simulink model "UDP_sensor_stream"  (R2021a)
settings: Solver=ode3  StartTime=0.0  StopTime=10.0  RelTol=1e-3
libraries: androidsensorlib x8, androidcommunicationlib x1
PreSaveFcn:
  | set_param(gcs, 'Location',[35 56 895 700 ])
settings Model: ExtModeTrigDuration=100  Creator=The MathWorks, Inc.  LastModifiedBy=shrey
settings SolverCC: AlgebraicLoopSolver=TrustRegion
settings DataIOCC: LimitDataPoints=on  SaveFormat=Array  ReturnWorkspaceOutputs=off
settings OptimizationCC: LifeSpan=1  MaxStackSize=64
settings DebuggingCC: UnderspecifiedInitializationDetection=Classic  MergeDetectMultiDrivingBlocksExec=none  ParameterPrecisionLossMsg=none  AllowSymbolicDim=off  SFUnexpectedBacktrackingDiag=warning  SFNoUnconditionalDefaultTransitionDiag=warning  SFExecutionAtInitializationDiag=none  SFMachineParentedDataDiag=warning  ArithmeticOperatorsInVariantConditions=warning
settings HardwareCC: ProdBitPerPointer=32  ProdBitPerSizeT=32  ProdBitPerPtrDiffT=32  ProdLargestAtomicInteger=Long  ProdLargestAtomicFloat=Double  ProdWordSize=32  ProdHWDeviceType=ARM Compatible->ARM Cortex  TargetLargestAtomicInteger=Long  TargetLargestAtomicFloat=Double  TargetEndianess=LittleEndian  TargetHWDeviceType=ARM Compatible->ARM Cortex  UseEmbeddedCoderFeatures=off  UseSimulinkCoderFeatures=off
settings ModelReferenceCC: PropagateSignalLabelsOutOfModel=off
settings SFSimCC: SimUseLocalCustomCode=off  CustomCodeUndefinedFunction=UseInterfaceOnly
settings RTWCC: SystemTargetFile=ert.tlc  HardwareBoard=Android Device  TemplateMakefile=ert_default_tmf  GenerateReport=on  RTWVerbose=off  RTWUseLocalCustomCode=off  Toolchain=Android SDK/NDK Tools  LaunchReport=on
settings CodeAppCC: ForceParamTrailComments=on  OperatorAnnotations=on  StateflowObjectComments=on  MATLABSourceComments=on
settings ERTTargetCC: MultiwordLength=2048  ERTCustomFileBanners=off  SupportContinuousTime=on  SupportNonInlinedSFcns=on  RemoveResetFunc=off  ModelStepFunctionPrototypeControlCompliant=off
settings ConfigComp: CovMetricSettings=dw  CovSaveCumulativeToWorkspaceVar=on  CovSaveSingleToWorkspaceVar=on  CovExternalEMLEnable=off  CovSFcnEnable=off

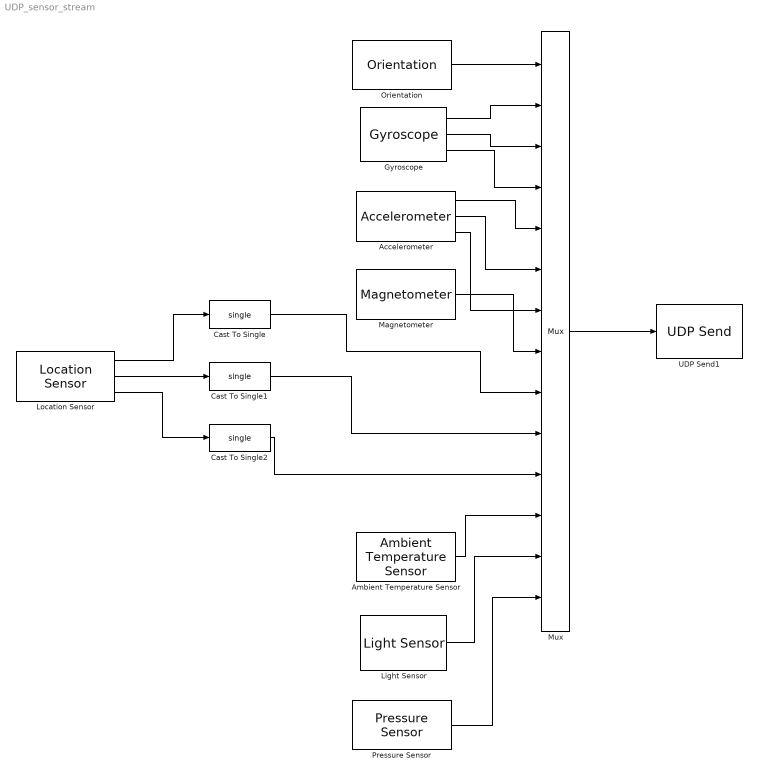
== system UDP_sensor_stream ==
  Accelerometer : androidsensorlib/Accelerometer  OutputVector=off  SampleTime=0.1  BlockPlatform=Android
      settings: SourceProductBaseCode=ANDROID
  Ambient Temperature Sensor : androidsensorlib/Ambient Temperature Sensor  SampleTime=0.1  BlockPlatform=Android
      settings: SourceProductBaseCode=ANDROID
  Cast To Single : DataTypeConversion  OutDataTypeStr=single
  Cast To Single1 : DataTypeConversion  OutDataTypeStr=single
  Cast To Single2 : DataTypeConversion  OutDataTypeStr=single
  Gyroscope : androidsensorlib/Gyroscope  OutputVector=off  SampleTime=2  BlockPlatform=Android
      settings: SourceProductBaseCode=ANDROID
  Light Sensor : androidsensorlib/Light Sensor  SampleTime=2  BlockPlatform=Android
      settings: SourceProductBaseCode=ANDROID
  Location Sensor : androidsensorlib/Location Sensor  OutputVector=off  SampleTime=0.1  BlockPlatform=Android
      settings: SourceProductBaseCode=ANDROID
  Magnetometer : androidsensorlib/Magnetometer  SampleTime=0.1
      settings: SourceProductBaseCode=ANDROID
  Mux : Mux  Inputs=14
  Orientation : androidsensorlib/Orientation  SampleTime=0.1
      settings: SourceProductBaseCode=ANDROID
  Pressure Sensor : androidsensorlib/Pressure Sensor  SampleTime=0.1  BlockPlatform=Android
      settings: SourceProductBaseCode=ANDROID
  UDP Send1 : androidcommunicationlib/UDP Send  remoteURL='192.168.1.104'  remotePort=20001  localURL='0.0.0.0'  localPortSource=Automatically determine  localPort=-1  sampletime=-1  blockPlatform=Android  separateLengthPort=0
      settings: SourceProductBaseCode=ANDROID
  wires:
  Mux/1 -> UDP Send1/1
  Orientation/1 -> Mux/1
  Gyroscope/1 -> Mux/2
  Gyroscope/2 -> Mux/3
  Gyroscope/3 -> Mux/4
  Accelerometer/1 -> Mux/5
  Accelerometer/2 -> Mux/6
  Accelerometer/3 -> Mux/7
  Magnetometer/1 -> Mux/8
  Location Sensor/2 -> Cast To Single1/1
  Location Sensor/3 -> Cast To Single2/1
  Ambient Temperature Sensor/1 -> Mux/12
  Light Sensor/1 -> Mux/13
  Pressure Sensor/1 -> Mux/14
  Location Sensor/1 -> Cast To Single/1
  Cast To Single/1 -> Mux/9
  Cast To Single1/1 -> Mux/10
  Cast To Single2/1 -> Mux/11
